simulink model "derivative"  (Simulink 6.5)
settings: Solver=ode4  StartTime=0.0  StopTime=10.0  FixedStep=0.1  RelTol=1e-3
settings Model: Creator=vjoel  LastModifiedBy=vjoel

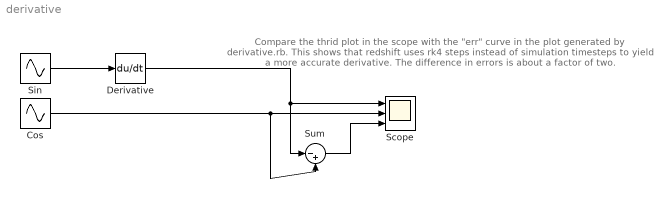
== system derivative ==
  note: Compare the thrid plot in the scope with the
      | "err" curve in the plot generated by derivative.rb.
      | This shows that redshift uses rk4 steps instead of simulation
      | timesteps to yield a more accurate derivative.
      | The difference in errors is about a factor of two.
  Cos : Sin  Phase=pi/2  SampleTime=0
  Derivative : Derivative
  Scope : Scope  NumInputPorts=3
      settings: YMin=-5~-5~-5  YMax=5~5~5
  Sin : Sin  SampleTime=0
  Sum : Sum  Inputs=|-+
  wires:
  Sin/1 -> Derivative/1
  Derivative/1 -> Scope/1, Sum/1
  Cos/1 -> Scope/2, Sum/2
  Sum/1 -> Scope/3
